simulink model "pll2"  (R2014a)
settings: Solver=ode45  StartTime=0.0  StopTime=0.3e-3  RelTol=1e-3
values from neighbouring files (symbols this model uses):
  Ci = 25e-12    (= 2.5e-11)    [pll_parameters.m]
  Cp1 = 6.3e-12    [pll_parameters.m]
  Cp3 = 2e-12    [pll_parameters.m]
  f0 = 26.93e9    (= 26930000000)    [pll_parameters.m]
  fref = 27e6    (= 27000000)    [pll_parameters.m]
  Iidn = -10.1e-6    (= -1.01e-05)    [pll_parameters.m]
  Iiup = 10.1e-6    (= 1.01e-05)    [pll_parameters.m]
  Ipdn = -505e-6    (= -0.000505)    [pll_parameters.m]
  Ipup = 505e-6    (= 0.000505)    [pll_parameters.m]
  Ki = 200e6    (= 200000000)    [pll_parameters.m]
  Kp = 25e6    (= 25000000)    [pll_parameters.m]
  N = 1000    [pll_parameters.m]
  phiref0 = 0    [pll_parameters.m]
  phiv0 = -0.4*2*pi    (= -2.51327412287)    [pll_parameters.m]
  Rp2 = 50e3    (= 50000)    [pll_parameters.m]
  Rp3 = 8e3    (= 8000)    [pll_parameters.m]
  td = 50e-12    (= 5e-11)    [pll_parameters.m]
  vi0 = 0.35    [pll_parameters.m]
  vp0 = 0    [pll_parameters.m]
  vp10 = 0    [pll_parameters.m]
libraries: simulink x1
settings Model: Creator=OmarAli  LastModifiedBy=OmarAli

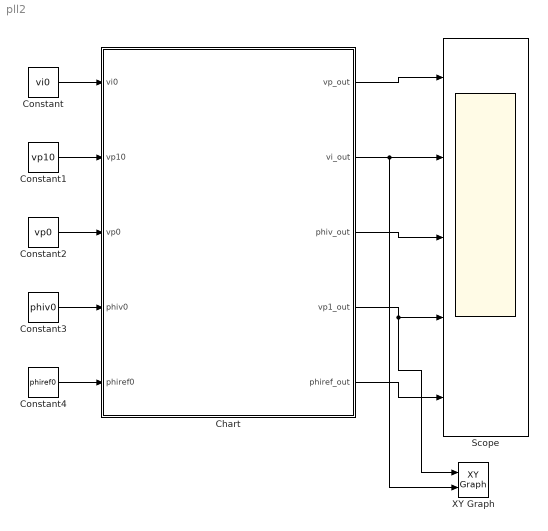
== system pll2 ==
  Chart : Stateflow chart  TreatAsAtomicUnit=on
  Constant : Constant  Value=vi0
  Constant1 : Constant  Value=vp10
  Constant2 : Constant  Value=vp0
  Constant3 : Constant  Value=phiv0
  Constant4 : Constant  Value=phiref0
  Scope : Scope  NumInputPorts=5
      settings: ShowLegends=on  YMin=-3~0~-3~-3~-2  YMax=5~3.5~7~4~7
  XY Graph : simulink/Sinks/XY Graph  xmin=-5  xmax=5  ymin=-5  ymax=5  st=-1
  wires:
  Constant/1 -> Chart/1(vi0)
  Constant1/1 -> Chart/2(vp10)
  Constant2/1 -> Chart/3(vp0)
  Constant3/1 -> Chart/4(phiv0)
  Constant4/1 -> Chart/5(phiref0)
  Chart/1(vp_out) -> Scope/1
  Chart/2(vi_out) -> XY Graph/2, Scope/2
  Chart/3(phiv_out) -> Scope/3
  Chart/4(vp1_out) -> XY Graph/1, Scope/4
  Chart/5(phiref_out) -> Scope/5

== stateflow chart pll2/Chart ==
  settings: updateMethod=CONTINUOUS
  state both_0
    du:
    vi_dot = 0;
    vp1_dot = -1*( vp1/Cp1)*(1/Rp2 + 1/Rp3) + vp/(Cp1 * Rp3);
    vp_dot = vp1/(Cp3*Rp3) - vp/(Cp3 * Rp3);
    phiv_dot = vi*Ki/N + vp * Kp/N + 2*pi* f0/N;
    phiref_dot = 2*pi*fref;
    t_dot = 1;
    vi_out = vi;
    vp1_out = vp1;
    vp_out = vp;
    phiv_out = phiv;
    phiref_out = phiref;
  state up_1
    du:
    vi_dot = Iiup/Ci;
    vp1_dot = -1*( vp1/Cp1)*(1/Rp2 + 1/Rp3) + vp/(Cp1 * Rp3);
    vp_dot = vp1/(Cp3*Rp3) - vp/(Cp3 * Rp3) + Ipup / Cp1;
    phiv_dot = vi*Ki/N + vp * Kp/N + 2*pi* f0/N;
    phiref_dot = 2*pi*fref;
    t_dot = 1;
    vi_out = vi;
    vp1_out = vp1;
    vp_out = vp;
    phiv_out = phiv;
    phiref_out = phiref;
  state dn_1
    du:
    vi_dot = Iidn/Ci;
    vp1_dot = -1*( vp1/Cp1)*(1/Rp2 + 1/Rp3) + vp/(Cp1 * Rp3);
    vp_dot = vp1/(Cp3*Rp3) - vp/(Cp3 * Rp3) + Ipdn / Cp1;
    phiv_dot = vi*Ki/N + vp * Kp/N + 2*pi* f0/N;
    phiref_dot = 2*pi*fref;
    t_dot = 1;
    vi_out = vi;
    vp1_out = vp1;
    vp_out = vp;
    phiv_out = phiv;
    phiref_out = phiref;
  state both_1
    du:
    vi_dot = (Iiup+Iidn)/Ci;
    vp1_dot = -1*( vp1/Cp1)*(1/Rp2 + 1/Rp3) + vp/(Cp1 * Rp3);
    vp_dot = vp1/(Cp3*Rp3) - vp/(Cp3 * Rp3) +  (Ipup+Ipdn) / Cp1;
    phiv_dot = vi*Ki/N + vp * Kp/N + 2*pi* f0/N;
    phiref_dot = 2*pi*fref;
    t_dot = 1;
    vi_out = vi;
    vp1_out = vp1;
    vp_out = vp;
    phiv_out = phiv;
    phiref_out = phiref;
  (default) -> both_0 : {vi = vi0;
      | vp1 = vp10;
      | vp = vp0;
      | phiv = phiv0;
      | phiref = phiref0;}
  both_0 -> up_1 [order 2] : [phiref >= 2*pi]
      | {phiv = phiv - 2*pi;
      | phiref = 0;}
  both_0 -> dn_1 [order 1] : [phiv>= 2*pi]
      | {phiref = phiref - 2*pi;
      | phiv = 0;}
  both_1 -> both_0 : [t >= td]
      | {t = 0;}
  up_1 -> both_1 : [phiv >= 0]
      | {t = 0;}
  dn_1 -> both_1 : [phiref >= 0]
      | {t= 0;}
  data: Cp3 parameter double =Cp3; Ki parameter double =Ki; vi local; Kp parameter double =Kp; vp1 local; Cp1 parameter double =Cp1; Rp2 parameter double =Rp2; Rp3 parameter double =Rp3; vp local; f0 parameter double =f0; fref parameter double =fref; Iiup parameter double =Iiup; Ci parameter double =Ci; Ipup parameter double =Ipup; Ipdn parameter double =Ipdn; Iidn parameter double =Iidn; td parameter double =td; vp_out output double; vi_out output double; phiv_out output double; vp1_out output double; phiref_out output double; phiv local; phiref local; t local; N parameter double =N; vi0 input double; vp10 input double; vp0 input double; phiv0 input double; phiref0 input double
  data vi settings: updateMethod=SF_CONTINUOUS_TIME_DATA
  data vp1 settings: updateMethod=SF_CONTINUOUS_TIME_DATA
  data vp settings: updateMethod=SF_CONTINUOUS_TIME_DATA
  data phiv settings: updateMethod=SF_CONTINUOUS_TIME_DATA
  data phiref settings: updateMethod=SF_CONTINUOUS_TIME_DATA
  data t settings: updateMethod=SF_CONTINUOUS_TIME_DATA
